simulink model "task_1"  (R2024a)
settings: Solver=VariableStepAuto  StartTime=0.0  StopTime=5  FixedStep=1e-5  MaxStep=0.1  RelTol=1e-5
undefined symbols (not defined in the file): a0, a1, idy, iy, u_num
settings Model: Creator=kit  LastModifiedBy=kit

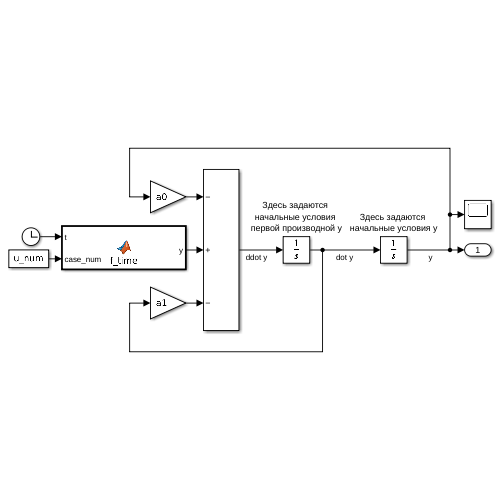
[thumbnail: Simulink's stored preview of the top-level diagram]
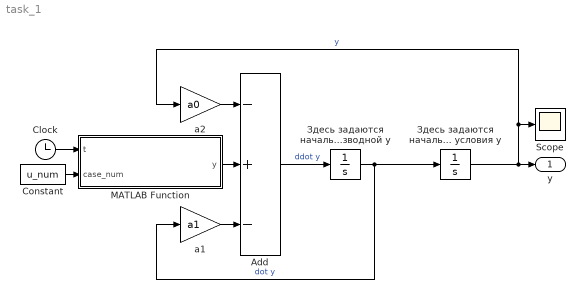
== system task_1 ==
  Add : Sum  Inputs=-+-
  Clock : Clock
  Constant : Constant  Value=u_num
  MATLAB Function : MATLAB Function  TreatAsAtomicUnit=on
  Scope : Scope
  a1 : Gain  Gain=a1
  a2 : Gain  Gain=a0
  Здесь задаются начальные условия первой производной y : Integrator  InitialCondition=idy
  Здесь задаются начальные условия y : Integrator  InitialCondition=iy
  y : Outport
  wires:
  Clock/1 -> MATLAB Function/1(t)
  MATLAB Function/1(y) -> Add/2
  a2/1 -> Add/1
  a1/1 -> Add/3
  Здесь задаются начальные условия первой производной y/1 -> Здесь задаются начальные условия y/1, a1/1  "dot y"
  Add/1 -> Здесь задаются начальные условия первой производной y/1  "ddot y"
  Здесь задаются начальные условия y/1 -> a2/1, Scope/1, y/1  "y"
  Constant/1 -> MATLAB Function/2(case_num)

== matlab function task_1/MATLAB Function ==
  data: t input; y output; case_num input
function y = f_time(t, case_num)
% case_num определяет, какую функцию использовать
    switch case_num
        case 1
            y = 2.5;
        case 2
            y = 0.8*t;
        case 3
            y = sin(8*t);
        otherwise
            y = 0; % На всякий случай
    end
end
